simulink model "ssc_lithium_cell_1RC_estim"  (R2017a)
settings: Solver=ode15s  StartTime=0  StopTime=37000  MaxStep=250  RelTol=1e-3  EnableMultiTasking=on
PreLoadFcn:
  | ssc_lithium_cell_1RC_estim_ini
undefined symbols (not defined in the file or in its folder): Capacity
libraries: nesl_utility x4, LiBatteryElements_lib x4, fl_lib x3
settings Model: Creator=psanghvi  LastModifiedBy=jgazzarr
settings DataIOCC: ExternalInput=[PulseData.time PulseData.current PulseData.voltage]  LoadExternalInput=on  SaveFormat=Array  SignalLogging=off  DSMLogging=off
settings OptimizationCC: EnhancedBackFolding=on  ExpressionDepthLimit=2147483647  LifeSpan=1  SimCompilerOptimization=on
settings DebuggingCC: UnderspecifiedInitializationDetection=Classic  MergeDetectMultiDrivingBlocksExec=none  SolverPrmCheckMsg=warning  FcnCallInpInsideContextMsg=warning  StateNameClashWarn=warning  SFUnexpectedBacktrackingDiag=warning  SFNoUnconditionalDefaultTransitionDiag=warning  SFExecutionAtInitializationDiag=none
settings HardwareCC: ProdBitPerPointer=32  ProdBitPerSizeT=32  ProdBitPerPtrDiffT=32  ProdLargestAtomicFloat=None  ProdIntDivRoundTo=Undefined  ProdEndianess=Unspecified  ProdWordSize=32  ProdHWDeviceType=32-bit Generic
settings ModelReferenceCC: PropagateSignalLabelsOutOfModel=off
settings SFSimCC: MATLABDynamicMemAlloc=off
settings RTWCC: SystemTargetFile=ert.tlc  GenCodeOnly=on  TemplateMakefile=ert_default_tmf  Description=Embedded Coder  GenerateReport=on  IncludeHyperlinkInReport=on  LaunchReport=on  GenerateTraceInfo=on  GenerateTraceReport=on  GenerateTraceReportSl=on  GenerateTraceReportSf=on  GenerateTraceReportEml=on
settings CodeAppCC: IgnoreCustomStorageClasses=off  CustomSymbolStrType=$N$R$M  InternalIdentifier=Classic
settings ERTTargetCC: MultiwordLength=2048  GenerateSampleERTMain=on  ERTCustomFileTemplate=example_file_process.tlc  ConvertIfToSwitch=off  SuppressUnreachableDefaultCases=off
settings ConfigComp: CovMetricSettings=dw  CovHtmlReporting=on  CovSaveCumulativeToWorkspaceVar=on  CovSaveSingleToWorkspaceVar=on  CovExternalEMLEnable=off

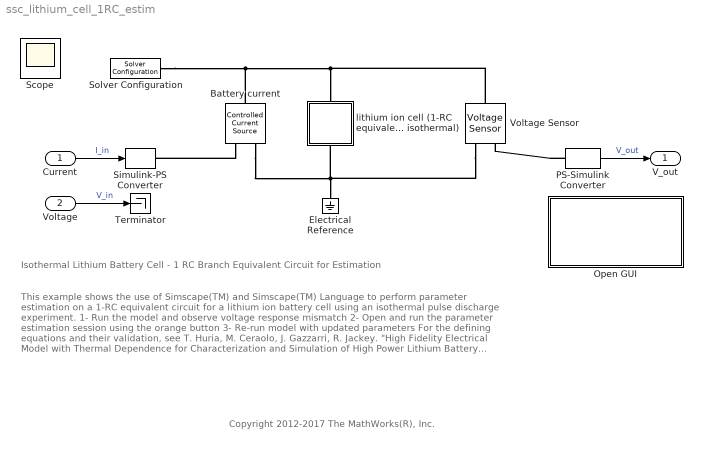
== system ssc_lithium_cell_1RC_estim ==
  note: Isothermal Lithium Battery Cell - 1 RC Branch Equivalent Circuit for Estimation
  note: This example shows the use of Simscape(TM) and Simscape(TM) Language to perform parameter estimation on a 1-RC equivalent circuit for a lithium ion battery cell using an isothermal pulse discharge experiment.
      | 1- Run the model and observe voltage response mismatch
      | 2- Open and run the parameter estimation session using the orange button
      | 3- Re-run model with updated parameters
      |
      | For the defining equations and their validation, see T. Huria, M. Ceraolo, J. Gazzarri, R. Jackey. "High Fidelity Electrical Model with
      | Thermal Dependence for Characterization and Simulation of High Power Lithium Battery Cells," IEEE International Electric Vehicle Conference,
      | March 2012.
  note: Copyright 2012-2017 The MathWorks(R), Inc.
  Current : Inport
  Voltage : Inport  Port=2
  Battery current : fl_lib/Electrical/Electrical Sources/Controlled Current Source
  Electrical Reference : fl_lib/Electrical/Electrical Elements/Electrical Reference
  Open GUI : Subsystem
      settings: OpenFcn=|
      | % speload('ssc_lithium_cell_SDO_Project', 'Project - ssc_lithium_cell_1RC_estim', 'One Temp Estim');
      | speload('ssc_lithium_cell_1RC_estim_spesession')
      mask Display: disp('Double click here\nto open the\nParameter Estimation\nApp with preloaded data')
  PS-Simulink Converter : nesl_utility/PS-Simulink Converter  PhysicalDomain=network_engine_domain  SubClassName=ps_output  LeftPortType=input  RightPortType=output  PseudoPeriodic=off  Frequencies=[]  Unit=V  AffineConversion=off
  Simulink-PS Converter : nesl_utility/Simulink-PS Converter  PhysicalDomain=network_engine_domain  SubClassName=ps_input  LeftPortType=input  RightPortType=output  PseudoPeriodic=off  Frequencies=[]  NoiseDistribution=none  NoiseParameters=[]  Unit=A  AffineConversion=off  FilteringAndDerivatives=zero  SimscapeFilterOrder=1  InputFilterTimeConstant=.001  UdotUserProvided=0
  Solver Configuration : nesl_utility/Solver Configuration  PhysicalDomain=network_engine_domain  SubClassName=solver  LeftPortType=input  RightPortType=generic  Accelerate=off  Tones=[]  Harmonics=[]  SimulateNoise=off  Profile=off  UseLocalSampling=off  EnableSwitchedLinearOptims=on  FrequencyDomain=off  UseCCode=off  RelTol=0.001  AbsTol=1e-06  MinStep=1e-09  ToWorkspace=off  RevertToSquareIcSolve=off  NumHomotopyIterations=100  PhasorMode=off  PhasorModeNumHarmonics=1  OverrideAbsTol=off  DoDC=off  ResidualTolerance=1e-9  UseLocalSolver=off  LocalSolverChoice=NE_BACKWARD_EULER_ADVANCER  LocalSolverSampleTime=.001  DoFixedCost=off  MaxNonlinIter=12  MaxModeIter=2  LinearAlgebra=Sparse  DelaysMemoryBudget=1024  AutomaticFiltering=on  FilteringTimeConstant=0.001
  Terminator : Terminator
  Voltage Sensor : fl_lib/Electrical/Electrical Sensors/Voltage Sensor
  "lithium ion cell (1-RC equivalent circuit model, isothermal)" : Subsystem
  V_out : Outport
  Scope : Scope
  wires:
  PS-Simulink Converter/1 -> V_out/1  "V_out"
  Current/1 -> Simulink-PS Converter/1  "I_in"
  Voltage/1 -> Terminator/1  "V_in"
  connections:
  Battery current/RConn1 -- Simulink-PS Converter/RConn1
  Battery current/LConn1 -- "lithium ion cell (1-RC equivalent circuit model, isothermal)"/LConn1 -- Voltage Sensor/LConn1 -- Solver Configuration/RConn1
  PS-Simulink Converter/LConn1 -- Voltage Sensor/RConn1
  Voltage Sensor/RConn2 -- Electrical Reference/LConn1 -- Battery current/RConn2 -- "lithium ion cell (1-RC equivalent circuit model, isothermal)"/RConn1

== system ssc_lithium_cell_1RC_estim/Open GUI ==

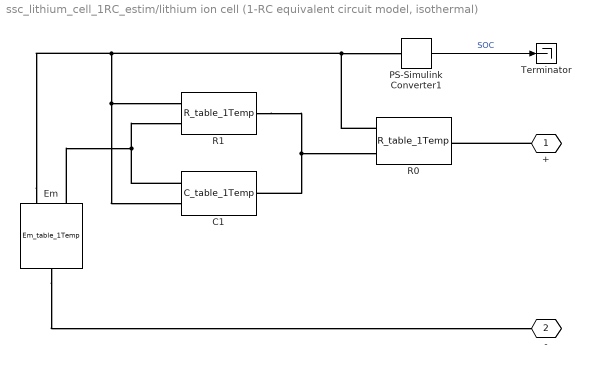
== system ssc_lithium_cell_1RC_estim/lithium ion cell (1-RC equivalent circuit model, isothermal) ==
  C1 : LiBatteryElements_lib/C_table_1Temp  C_Table=C1 F  SOC_Table=SOC_LUT  v0=0 V  mask(C_table_1Temp){}
      mask Display: image('C_fig.png');
  Em : LiBatteryElements_lib/Em_table_1Temp  Em_Table=Em V  SOC_Table=SOC_LUT  C=Capacity hr*A  Qinit=Qe_init hr*A  mask(Em_table_1Temp){}
      mask Display: image('V_fig.png');
  PS-Simulink Converter1 : nesl_utility/PS-Simulink Converter  PhysicalDomain=network_engine_domain  SubClassName=ps_output  LeftPortType=input  RightPortType=output  PseudoPeriodic=off  Frequencies=[]  Unit=1  AffineConversion=off
  R0 : LiBatteryElements_lib/R_table_1Temp  R_Table=R0 Ohm  SOC_Table=SOC_LUT  mask(R_table_1Temp){}
      mask Display: image('R_fig.png');
  R1 : LiBatteryElements_lib/R_table_1Temp  R_Table=R1 Ohm  SOC_Table=SOC_LUT  mask(R_table_1Temp){}
      mask Display: image('R_fig.png');
  Terminator : Terminator
  + : PMIOPort  Tag=PMCPort  Port=1  Side=Left
  - : PMIOPort  Tag=PMCPort  Port=2  Side=Right
  wires:
  PS-Simulink Converter1/1 -> Terminator/1  "SOC"
  connections:
  Em/LConn1 -- C1/LConn1 -- R1/LConn1
  +/RConn1 -- R0/RConn1
  Em/RConn1 -- -/RConn1
  Em/LConn2 -- C1/LConn2 -- R1/LConn2 -- PS-Simulink Converter1/LConn1 -- R0/LConn2
  R1/RConn1 -- C1/RConn1 -- R0/LConn1
